simulink model "Clustering2Tanques"  (R2019a)
settings: Solver=VariableStepAuto  StartTime=0.0  StopTime=8000  RelTol=1e-3
values from neighbouring files (symbols this model uses):
  al = 95.52    [parametros.m]
  am = 64    [parametros.m]
  klm = 0.9580    (= 0.958)    [parametros.m]
  kr = 1.8    [parametros.m]
  Nivel2_err = 0    [parametros.m]
  Nivel_err = 0    [parametros.m]
  Tuberia_err = 0    [parametros.m]
settings Model: Creator=jalil  LastModifiedBy=david
settings DebuggingCC: PregeneratedLibrarySubsystemCodeDiagnostic=none  ArithmeticOperatorsInVariantConditions=warning

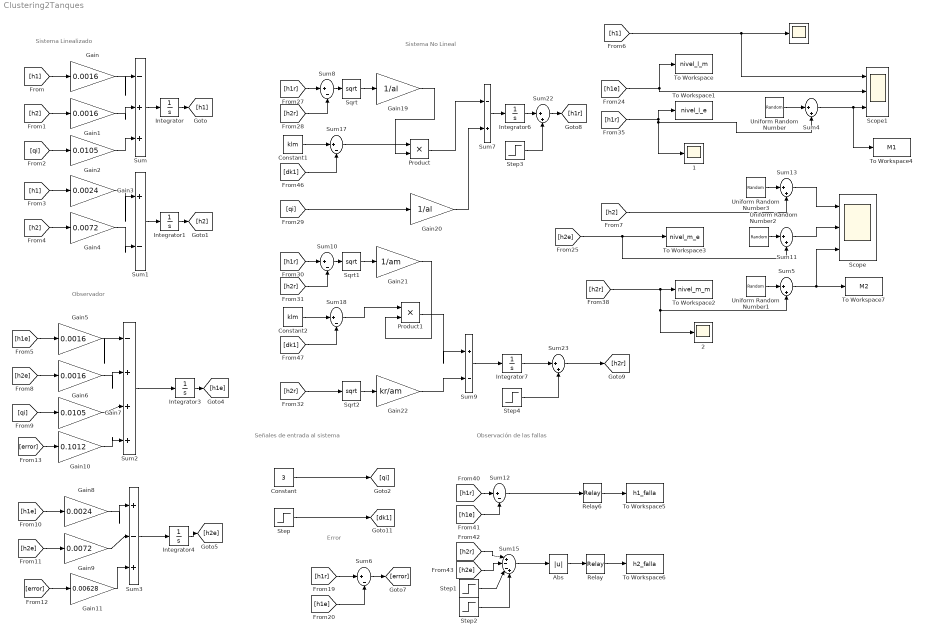
== system Clustering2Tanques ==
  note: Observador
  note: Sistema No Lineal
  note: Sistema Linealizado
  note: Señales de entrada al sistema
  note: Error
  note: Observación de las fallas
  " " : Scope
  " 1" : Scope
  " 2" : Scope
  Abs : Abs
  Constant : Constant  Value=3
  Constant1 : Constant  Value=klm
  Constant2 : Constant  Value=klm
  Gain{,1,5..6} (4 alike) : Gain  Gain=0.0016
  Gain10 : Gain  Gain=0.1012
  Gain11 : Gain  Gain=0.00628
  Gain19 : Gain  Gain=1/al
  Gain2 : Gain  Gain=0.0105
  Gain20 : Gain  Gain=1/al
  Gain21 : Gain  Gain=1/am
  Gain22 : Gain  Gain=kr/am
  Gain3 : Gain  Gain=0.0024
  Gain4 : Gain  Gain=0.0072
  Gain7 : Gain  Gain=0.0105
  Gain8 : Gain  Gain=0.0024
  Gain9 : Gain  Gain=0.0072
  Integrator{,1,6..7} (4 alike) : Integrator
  Integrator3 : Integrator  InitialCondition=1
  Integrator4 : Integrator  InitialCondition=-1
  Product : Product
  Product1 : Product
  Relay : Relay  OnSwitchValue=1  OffSwitchValue=-1000
  Relay6 : Relay  OnSwitchValue=1.5  OffSwitchValue=-1000
  Scope : Scope  NumInputPorts=3
  Scope1 : Scope  NumInputPorts=3
  Sqrt : Sqrt  SaturateOnIntegerOverflow=on
  Sqrt1 : Sqrt  SaturateOnIntegerOverflow=on
  Sqrt2 : Sqrt  SaturateOnIntegerOverflow=on
  Step : Step  Time=4000  After=Tuberia_err  SampleTime=0
  Step1 : Step  Time=300  After=-0.6  SampleTime=0
  Step2 : Step  Time=300  After=0.6  SampleTime=0
  Step3 : Step  Time=4000  After=Nivel_err  SampleTime=0
  Step4 : Step  Time=4000  After=Nivel2_err  SampleTime=0
  Sum : Sum  Inputs=|-++
  Sum{1,6,8..10,12,17..18} (8 alike) : Sum  Inputs=|+-
  Sum{4..5,11,13,22..23} (6 alike) : Sum  Inputs=|++
  Sum15 : Sum  Inputs=|+--+
  Sum2 : Sum  Inputs=|-+++
  Sum3 : Sum  Inputs=|+-+
  Sum7 : Sum  Inputs=|-+
  To Workspace : ToWorkspace  VariableName=nivel_l_m  SaveFormat=Timeseries  SampleTime=-1
  To Workspace1 : ToWorkspace  VariableName=nivel_l_e  SaveFormat=Timeseries  SampleTime=-1
  To Workspace2 : ToWorkspace  VariableName=nivel_m_m  SaveFormat=Timeseries  SampleTime=-1
  To Workspace3 : ToWorkspace  VariableName=nivel_m_e  SaveFormat=Timeseries  SampleTime=-1
  To Workspace4 : ToWorkspace  VariableName=M1  SaveFormat=Timeseries  SampleTime=-1
      settings: Save2DSignal=2-D array (concatenate along first dimension)
  To Workspace5 : ToWorkspace  VariableName=h1_falla  SaveFormat=Timeseries  SampleTime=-1
  To Workspace6 : ToWorkspace  VariableName=h2_falla  SaveFormat=Timeseries  SampleTime=-1
  To Workspace7 : ToWorkspace  VariableName=M2  SaveFormat=Timeseries  SampleTime=-1
      settings: Save2DSignal=2-D array (concatenate along first dimension)
  Uniform Random Number : UniformRandomNumber  Minimum=-3  Maximum=3
  Uniform Random Number1 : UniformRandomNumber  Minimum=-3  Maximum=3  SampleTime=1
  Uniform Random Number2 : UniformRandomNumber  Minimum=-3  Maximum=3  SampleTime=1
  Uniform Random Number3 : UniformRandomNumber  Minimum=-3  Maximum=3  SampleTime=1
  wires:
  [h1] -> Gain/1
  Gain/1 -> Sum/1
  [h2] -> Gain1/1
  Gain1/1 -> Sum/2
  [qi] -> Gain2/1
  Gain2/1 -> Sum/3
  Sum/1 -> Integrator/1
  Integrator/1 -> [h1]
  Integrator1/1 -> [h2]
  Sum1/1 -> Integrator1/1
  Gain4/1 -> Sum1/2
  [h2] -> Gain4/1
  Gain3/1 -> Sum1/1
  [h1] -> Gain3/1
  Constant/1 -> [qi]
  Integrator4/1 -> [h2e]
  Integrator3/1 -> [h1e]
  [h1r] -> Sum6/1
  [h1e] -> Sum6/2
  Sum6/1 -> [error]
  [h1e] -> Scope1/2, To Workspace/1
  Sum7/1 -> Integrator6/1
  [h2r] -> Sum8/2
  [h1r] -> Sum8/1
  Sum8/1 -> Sqrt/1
  Sqrt/1 -> Gain19/1
  [qi] -> Gain20/1
  Gain20/1 -> Sum7/2
  Sum9/1 -> Integrator7/1
  Sum10/1 -> Sqrt1/1
  [h2r] -> Sum10/2
  Sqrt1/1 -> Gain21/1
  [h1r] -> Sum10/1
  Sqrt2/1 -> Gain22/1
  [h1r] -> Sum4/2, " 1"/1, To Workspace1/1
  Constant1/1 -> Sum17/1
  [dk1] -> Sum17/2
  Sum17/1 -> Product/1
  Gain19/1 -> Product/2
  Product/1 -> Sum7/1
  Gain21/1 -> Product1/2
  Product1/1 -> Sum9/1
  Sum18/1 -> Product1/1
  [dk1] -> Sum18/2
  Constant2/1 -> Sum18/1
  Step/1 -> [dk1]
  Integrator6/1 -> Sum22/1
  Step3/1 -> Sum22/2
  Sum22/1 -> [h1r]
  Integrator7/1 -> Sum23/1
  Step4/1 -> Sum23/2
  Sum23/1 -> [h2r]
  [h1e] -> Gain8/1
  Gain6/1 -> Sum2/2
  [qi] -> Gain7/1
  Gain5/1 -> Sum2/1
  Gain8/1 -> Sum3/1
  [h2e] -> Gain6/1
  Gain7/1 -> Sum2/3
  [h2e] -> Gain9/1
  Sum2/1 -> Integrator3/1
  Sum3/1 -> Integrator4/1
  [h1e] -> Gain5/1
  Gain9/1 -> Sum3/2
  [error] -> Gain10/1
  Gain10/1 -> Sum2/4
  [error] -> Gain11/1
  Gain11/1 -> Sum3/3
  Gain22/1 -> Sum9/2
  [h2r] -> Sqrt2/1
  Step2/1 -> Sum15/4
  Abs/1 -> Relay/1
  [h2r] -> Sum15/1
  Step1/1 -> Sum15/3
  Sum15/1 -> Abs/1
  Relay6/1 -> To Workspace5/1
  [h1r] -> Sum12/1
  Relay/1 -> To Workspace6/1
  Sum12/1 -> Relay6/1
  [h1e] -> Sum12/2
  [h2e] -> Sum15/2
  [h2r] -> To Workspace2/1, Sum5/2, " 2"/1
  [h2e] -> To Workspace3/1, Sum11/2
  [h1] -> Scope1/1, " "/1
  Uniform Random Number/1 -> Sum4/1
  Sum4/1 -> To Workspace4/1, Scope1/3
  Sum5/1 -> To Workspace7/1, Scope/3
  Uniform Random Number1/1 -> Sum5/1
  Uniform Random Number2/1 -> Sum11/1
  Sum11/1 -> Scope/2
  Sum13/1 -> Scope/1
  Uniform Random Number3/1 -> Sum13/1
  [h2] -> Sum13/2
